simulink model "ResetScheme"  (R2013a)
settings: Solver=FixedStepDiscrete  StartTime=0.0  StopTime=CONFIG.SIMULATION_TIME  FixedStep=CONFIG.Ts  RelTol=1e-3
undefined symbols (not defined in the file or in its folder): starting_joint_pos
libraries: WBToolboxLibrary x1
settings Model: Creator=valerio  LastModifiedBy=valerio

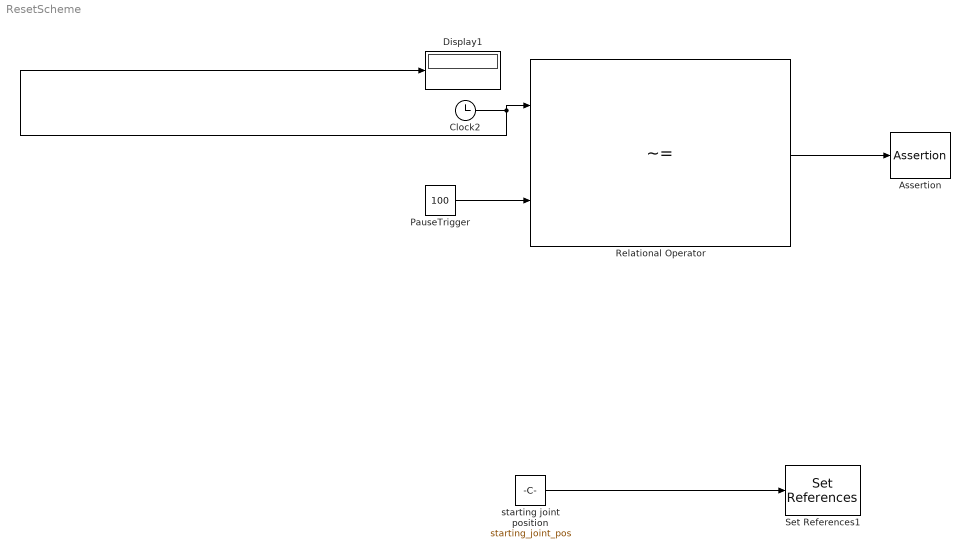
== system ResetScheme ==
  Assertion : Assertion  AssertionFailFcn=set_param(bdroot,'SimulationCommand','pause');finish_simulation=1;  StopWhenAssertionFail=off
  Clock2 : Clock
  Display1 : Display
  PauseTrigger : Constant  Value=100
  Relational Operator : RelationalOperator  Operator=~=  OutDataTypeStr=boolean
  Set References1 : WBToolboxLibrary/wholeBodyActuators/Set References  controlType=Position Direct  fullOrSubControl=Full  controlledJoints=''  robotName=WBT_robotName  localName=WBT_modelName  wbiFile=WBT_wbiFilename  wbiList=WBT_wbiList
  starting joint position : Constant  Value=starting_joint_pos
  wires:
  Clock2/1 -> Display1/1, Relational Operator/1
  Relational Operator/1 -> Assertion/1
  PauseTrigger/1 -> Relational Operator/2
  starting joint position/1 -> Set References1/1
